simulink subsystem "deadtime"  (R2022b)
settings: Solver=VariableStepAuto  StartTime=0.0  StopTime=10.0  RelTol=1e-3
libraries: spsEdgeDetectorLib x1
settings Model: Creator=jack  LastModifiedBy=jack

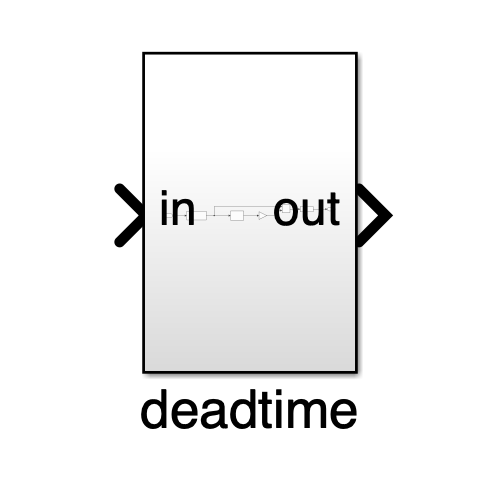
[thumbnail: Simulink's stored preview of the top-level diagram]
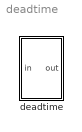
== system deadtime ==
  deadtime : Subsystem

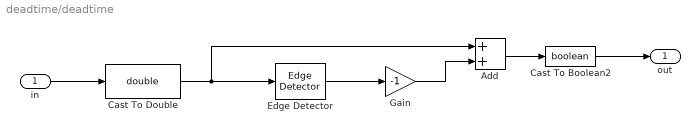
== system deadtime/deadtime ==
  in : Inport
  Add : Sum
  Cast To Boolean2 : DataTypeConversion  OutDataTypeStr=boolean  SaturateOnIntegerOverflow=off  RndMeth=Floor
  Cast To Double : DataTypeConversion  OutDataTypeStr=double  SaturateOnIntegerOverflow=off  RndMeth=Floor
  Edge Detector : spsEdgeDetectorLib/Edge Detector  model=Rising  ic=0  Ts=-1
      settings: LibrarySourceBlock=sps_lib/Control/Edge Detector
  Gain : Gain  Gain=-1
  out : Outport
  wires:
  in/1 -> Cast To Double/1
  Gain/1 -> Add/2
  Cast To Double/1 -> Add/1, Edge Detector/1
  Edge Detector/1 -> Gain/1
  Add/1 -> Cast To Boolean2/1
  Cast To Boolean2/1 -> out/1
